simulink model "EstimadorComAtraso"  (R2015a)
settings: Solver=ode45  StartTime=0.0  StopTime=10.0  RelTol=1e-3
settings Model: Creator=user  LastModifiedBy=user

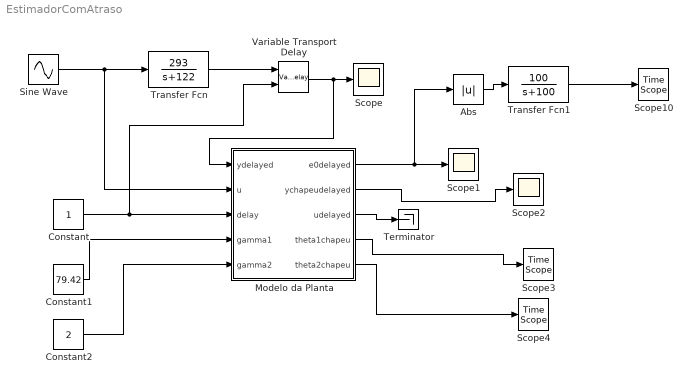
== system EstimadorComAtraso ==
  Abs : Abs
  Constant : Constant
  Constant1 : Constant  Value=79.42
  Constant2 : Constant  Value=2
  Modelo da Planta : Subsystem  Description=First Order Transfer Function Estimation Block
  Scope : Scope
      settings: SaveName=ScopeData5
  Scope1 : Scope
      settings: YMin=-111500  YMax=-105000
  Scope10 : TimeScope
  Scope2 : Scope
      settings: YMin=-0.75  YMax=0.75  SaveName=ScopeData2
  Scope3 : TimeScope
  Scope4 : TimeScope
  Sine Wave : Sin  Frequency=10  SampleTime=0
  Terminator : Terminator
  Transfer Fcn : TransferFcn  Numerator=[293]  Denominator=[1 122]
  Transfer Fcn1 : TransferFcn  Numerator=[100]  Denominator=[1 100]
  Variable Transport Delay : VariableTransportDelay  VariableDelayType=Variable transport delay  MaximumDelay=10  MaximumPoints=4096
  wires:
  Modelo da Planta/4(theta1chapeu) -> Scope3/1
  Modelo da Planta/1(e0delayed) -> Abs/1, Scope1/1
  Modelo da Planta/2(ychapeudelayed) -> Scope2/1
  Modelo da Planta/5(theta2chapeu) -> Scope4/1
  Constant/1 -> Variable Transport Delay/2, Modelo da Planta/3(delay)
  Constant1/1 -> Modelo da Planta/4(gamma1)
  Constant2/1 -> Modelo da Planta/5(gamma2)
  Transfer Fcn1/1 -> Scope10/1
  Abs/1 -> Transfer Fcn1/1
  Sine Wave/1 -> Modelo da Planta/2(u), Transfer Fcn/1
  Transfer Fcn/1 -> Variable Transport Delay/1
  Variable Transport Delay/1 -> Modelo da Planta/1(ydelayed), Scope/1
  Modelo da Planta/3(udelayed) -> Terminator/1

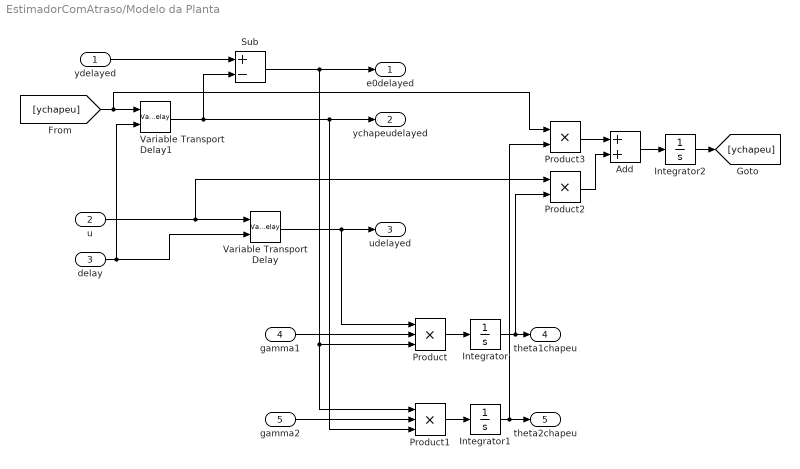
== system EstimadorComAtraso/Modelo da Planta ==
  ydelayed : Inport
  u : Inport  Port=2
  delay : Inport  Port=3
  gamma1 : Inport  Port=4
  gamma2 : Inport  Port=5
  Add : Sum
  Integrator : Integrator
  Integrator1 : Integrator
  Integrator2 : Integrator
  Product : Product  Inputs=3
  Product1 : Product  Inputs=3
  Product2 : Product
  Product3 : Product
  Sub : Sum  Inputs=+-
  Variable Transport Delay : VariableTransportDelay  VariableDelayType=Variable transport delay  MaximumDelay=10
  Variable Transport Delay1 : VariableTransportDelay  VariableDelayType=Variable transport delay  MaximumDelay=10
  e0delayed : Outport
  ychapeudelayed : Outport  Port=2
  udelayed : Outport  Port=3
  theta1chapeu : Outport  Port=4
  theta2chapeu : Outport  Port=5
  wires:
  ydelayed/1 -> Sub/1
  Sub/1 -> Product1/1, Product/3, e0delayed/1
  delay/1 -> Variable Transport Delay1/2, Variable Transport Delay/2
  u/1 -> Product2/1, Variable Transport Delay/1
  Variable Transport Delay/1 -> Product/1, udelayed/1
  gamma1/1 -> Product/2
  Product/1 -> Integrator/1
  Integrator/1 -> Product2/2, theta1chapeu/1
  gamma2/1 -> Product1/2
  [ychapeu] -> Product3/1, Variable Transport Delay1/1
  Variable Transport Delay1/1 -> Product1/3, ychapeudelayed/1, Sub/2
  Product1/1 -> Integrator1/1
  Integrator1/1 -> Product3/2, theta2chapeu/1
  Product3/1 -> Add/1
  Product2/1 -> Add/2
  Add/1 -> Integrator2/1
  Integrator2/1 -> [ychapeu]
